simulink model "flash_led"  (R2026a)
settings: Solver=FixedStepDiscrete  StopTime=50
model workspace (MAT data in the model file):
  MAX_COUNT = 5000000
libraries: hdlsllib x2
settings Model: DataTypeOverride=Off  Creator=KoayXianCong  LastModifiedBy=KoayXianCong
settings OptimizationCC: ConditionallyExecuteInputs=off  InheritOutputTypeSmallerThanSingle=on
settings DebuggingCC: ArtificialAlgebraicLoopMsg=error  SingleTaskRateTransMsg=error
settings HardwareCC: ProdHWDeviceType=ASIC/FPGA->ASIC/FPGA  TargetBitPerPointer=64.0  TargetBitPerSizeT=64.0  TargetBitPerPtrDiffT=64.0  TargetLongLongMode=on  TargetIntDivRoundTo=Zero  TargetEndianess=LittleEndian  TargetWordSize=64.0  TargetHWDeviceType=Custom Processor->MATLAB Host Computer  ProdEqTarget=off

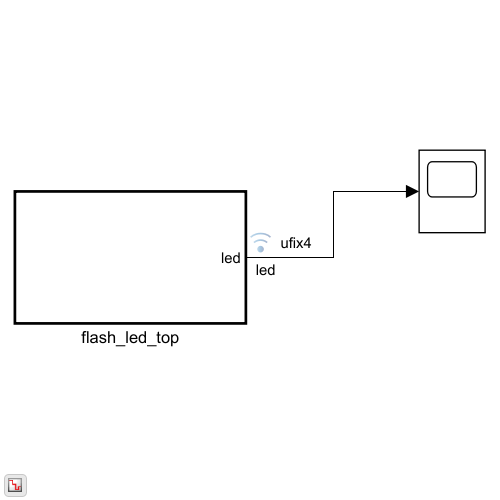
[thumbnail: Simulink's stored preview of the top-level diagram]
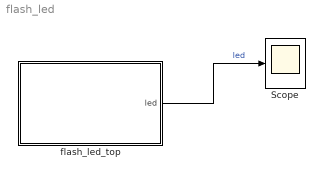
== system flash_led ==
  Scope : Scope
      settings: ActiveDisplayYMinimum=-1  ActiveDisplayYMaximum=1
  flash_led_top : Subsystem  TreatAsAtomicUnit=on
  wires:
  flash_led_top/1(led) -> Scope/1  "led"

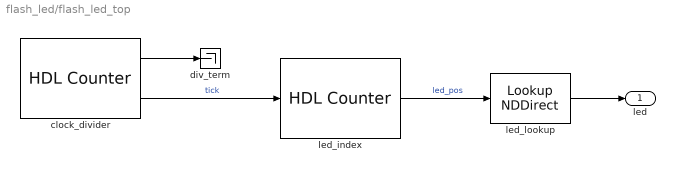
== system flash_led/flash_led_top ==
  clock_divider : hdlsllib/Sources/HDL Counter  CountType=Count limited  CountInit=0  CountStep=1  CountMax=MAX_COUNT-1  CountFromType=Initial value  CountFrom=0  CountResetPort=off  CountLoadPort=off  CountEnbPort=off  CountDirPort=off  CountHitOutputPort=on  CountDataType=Unsigned  CountWordLen=23  CountFracLen=0  CountSampTime=1
  div_term : Terminator
  led_index : hdlsllib/Sources/HDL Counter  CountType=Count limited  CountInit=0  CountStep=1  CountMax=3  CountFromType=Initial value  CountFrom=0  CountResetPort=off  CountLoadPort=off  CountEnbPort=on  CountDirPort=off  CountHitOutputPort=off  CountDataType=Unsigned  CountWordLen=2  CountFracLen=0  CountSampTime=1
  led_lookup : LookupNDDirect  NumberOfTableDimensions=1  Table=uint8([1 2 4 8])  TableDataTypeStr=fixdt(0,4,0)
  led : Outport
  wires:
  clock_divider/2 -> led_index/1  "tick"
  led_index/1 -> led_lookup/1  "led_pos"
  led_lookup/1 -> led/1
  clock_divider/1 -> div_term/1
